simulink model "Regler_opt"  (R2026a)
settings: Solver=ode23s  StartTime=tSim(1)  StopTime=tSim(end)  FixedStep=tStep  EnableMultiTasking=on
values from neighbouring files (symbols this model uses):
  A = [ 0,      1, 0,      0 ... (first row only)    [A4_4.m]    (also in reglerInit.m = [0, 1, 0, 0; reglerInit_fin.m = [0, 1, 0, 0; reglerInit_gain_scheduling.m = [0, 1, 0, 0; reglerInit_opt.m = [0, 1, 0, 0)
  A_grid = zeros(N_ml, 16)    [reglerInit_fin.m]    (also in reglerInit_opt1.m; reglerInit_opt2.m; reglerInit_opt3.m; reglerInit_opt4.m)
  a_lim_large = 3.0    (= 3)    [reglerInit_opt4.m]
  a_lim_medium = 2.6    [reglerInit_opt4.m]
  a_lim_small = 1.4    [reglerInit_opt4.m]
  A_obs = A - L_obs*C    [reglerInit.m]    (also in reglerInit_gain_scheduling.m; reglerInit_opt.m)
  a_ref0 = 0    [reglerInit_fin.m]    (also in reglerInit_opt2.m; reglerInit_opt3.m; reglerInit_opt4.m)
  a_ref_lim = 3.91175    [reglerInit_fin.m]    (also in reglerInit_opt2.m = 3.8; reglerInit_opt3.m = 3.8)
  A_traj = [0, 1, 0 ... (first row only)    [reglerInit_opt.m]    (also in reglerInit_opt1.m)
  B = [0; -30.49; 0; 30.49]    [A4_4.m]    (also in reglerInit.m; reglerInit_fin.m; reglerInit_gain_scheduling.m; reglerInit_opt.m)
  B_obs = [B, L_obs]    [reglerInit.m]    (also in reglerInit_gain_scheduling.m; reglerInit_opt.m)
  B_traj = [0 ... (first row only)    [reglerInit_opt.m]    (also in reglerInit_opt1.m)
  C = [1 0 0 0 ... (first row only)    [reglerInit.m]    (also in reglerInit_fin.m; reglerInit_gain_scheduling.m; reglerInit_opt.m; reglerInit_opt1.m)
  C_obs = eye(4)    [reglerInit.m]    (also in reglerInit_gain_scheduling.m; reglerInit_opt.m)
  C_traj = eye(3)    [reglerInit_opt.m]    (also in reglerInit_opt1.m)
  d_capture_full = 0.03    [reglerInit_opt3.m]    (also in reglerInit_opt4.m = 0.1)
  d_capture_start = 0.10    (= 0.1)    [reglerInit_opt3.m]    (also in reglerInit_opt4.m = 0.35)
  d_large = 1.18779    [reglerInit_fin.m]    (also in reglerInit_opt2.m = 1.3; reglerInit_opt3.m = 1.3; reglerInit_opt4.m = 1.2)
  D_obs = zeros(4,3)    [reglerInit.m]    (also in reglerInit_gain_scheduling.m; reglerInit_opt.m)
  d_small = 0.5719    [reglerInit_fin.m]    (also in reglerInit_opt2.m = 0.45; reglerInit_opt3.m = 0.45; reglerInit_opt4.m = 0.35)
  D_traj = zeros(3,1)    [reglerInit_opt.m]    (also in reglerInit_opt1.m)
  d_traj_capture = 0.35    [reglerInit_opt4.m]
  ff_gain = 0.942931    [reglerInit_fin.m]    (also in reglerInit_opt.m = 1; reglerInit_opt1.m = 1; reglerInit_opt2.m = 1; reglerInit_opt3.m = 1)
  g = 9.81    [reglerInit_fin.m]    (also in reglerInit_opt.m; reglerInit_opt1.m; reglerInit_opt2.m; reglerInit_opt3.m)
  gamma_phi = 0.195386    [reglerInit_fin.m]    (also in reglerInit_opt2.m = 0.3; reglerInit_opt3.m = 0.3; reglerInit_opt4.m = 0)
  j_lim_large = 14.0    (= 14)    [reglerInit_opt4.m]
  j_lim_medium = 12.0    (= 12)    [reglerInit_opt4.m]
  j_lim_small = 6.0    (= 6)    [reglerInit_opt4.m]
  j_ref_lim = 24.6332    [reglerInit_fin.m]    (also in reglerInit_opt2.m = 20; reglerInit_opt3.m = 20)
  K_capture_grid = zeros(N_ml, 4)    [reglerInit_opt3.m]    (also in reglerInit_opt4.m)
  K_drive_grid = zeros(N_ml, 4)    [reglerInit_opt3.m]    (also in reglerInit_opt4.m)
  K_grid = zeros(N_ml, 4)    [reglerInit_fin.m]    (also in reglerInit_opt1.m; reglerInit_opt2.m)
  K_lqr = lqr(A, B, Q_lqr, R_lqr)    [reglerInit_fin.m]    (also in reglerInit_opt.m; reglerInit_opt1.m; reglerInit_opt2.m; reglerInit_opt3.m)
  k_r = 7.2e-3    (= 0.0072)    [reglerInit_fin.m]    (also in reglerInit_opt.m; reglerInit_opt1.m; reglerInit_opt2.m; reglerInit_opt3.m)
  kd_traj_capture = 7.0    (= 7)    [reglerInit_opt4.m]
  kp_traj_capture = 16.0    (= 16)    [reglerInit_opt4.m]
  l = 1.0    (= 1)    [reglerInit_opt3.m]    (also in reglerInit_opt4.m)
  L_grid = zeros(N_ml, 8)    [reglerInit_fin.m]    (also in reglerInit_opt1.m; reglerInit_opt2.m; reglerInit_opt3.m; reglerInit_opt4.m)
  L_obs = place(A', C', obs_poles)'    [reglerInit.m]    (also in reglerInit_fin.m; reglerInit_gain_scheduling.m; reglerInit_opt.m; reglerInit_opt1.m)
  M_ff_max = 0.39    [reglerInit_fin.m]    (also in reglerInit_opt.m = 0.34; reglerInit_opt1.m = 0.34; reglerInit_opt2.m = 0.34; reglerInit_opt3.m = 0.34)
  M_max_total = 0.4    [reglerInit.m]    (also in reglerInit_fin.m; reglerInit_gain_scheduling.m; reglerInit_opt.m; reglerInit_opt1.m)
  m_s = 0.8    [reglerInit_fin.m]    (also in reglerInit_opt.m; reglerInit_opt1.m; reglerInit_opt2.m; reglerInit_opt3.m)
  ml_grid = linspace(1, 5, 17)    [reglerInit_fin.m]    (also in reglerInit_opt1.m; reglerInit_opt2.m; reglerInit_opt3.m; reglerInit_opt4.m)
  omega_ref_large = 2.08014    [reglerInit_fin.m]    (also in reglerInit_opt2.m = 2; reglerInit_opt3.m = 2)
  omega_ref_medium = 3.57058    [reglerInit_fin.m]    (also in reglerInit_opt2.m = 3.3; reglerInit_opt3.m = 3.3)
  omega_ref_small = 3.92272    [reglerInit_fin.m]    (also in reglerInit_opt2.m = 3.3; reglerInit_opt3.m = 3.3)
  phi_ref_lim = deg2rad(35)    [reglerInit_fin.m]    (also in reglerInit_opt2.m = deg2rad(18); reglerInit_opt3.m = deg2rad(18); reglerInit_opt4.m = deg2rad(10))
  phi_slow_1 = deg2rad(26.517)    [reglerInit_fin.m]    (also in reglerInit_opt2.m = deg2rad(28); reglerInit_opt3.m = deg2rad(28); reglerInit_opt4.m = deg2rad(28))
  phi_slow_2 = deg2rad(30.8674)    [reglerInit_fin.m]    (also in reglerInit_opt2.m = deg2rad(36); reglerInit_opt3.m = deg2rad(36); reglerInit_opt4.m = deg2rad(36))
  phidot_ref_lim = 1.6    [reglerInit_fin.m]    (also in reglerInit_opt2.m = 0.8; reglerInit_opt3.m = 0.8; reglerInit_opt4.m = 0)
  r_wheel = 0.041    [reglerInit_fin.m]    (also in reglerInit_opt.m; reglerInit_opt1.m; reglerInit_opt2.m; reglerInit_opt3.m)
  T_a_ref = 0.12    [reglerInit_opt4.m]
  v_lim_large = 2.3    [reglerInit_opt4.m]
  v_lim_medium = 1.8    [reglerInit_opt4.m]
  v_lim_small = 0.75    [reglerInit_opt4.m]
  v_ref0 = 0    [reglerInit_fin.m]    (also in reglerInit_opt2.m; reglerInit_opt3.m; reglerInit_opt4.m)
  x_ref0 = 0    [reglerInit_fin.m]    (also in reglerInit_opt2.m; reglerInit_opt3.m; reglerInit_opt4.m)
  xhat0 = [0, 0, 0, 0]    [reglerInit.m]    (also in reglerInit_fin.m = [0; 0; 0; 0]; reglerInit_gain_scheduling.m; reglerInit_opt.m = [0; 0; 0; 0]; reglerInit_opt1.m = [0; 0; 0; 0])
  xtraj0 = [0; 0; 0]    [reglerInit_opt.m]    (also in reglerInit_opt1.m)
settings Model: Creator=Henning Schlüter  LastModifiedBy=louis
settings DataIOCC: SignalLoggingSaveFormat=ModelDataLogs
settings DebuggingCC: UnderspecifiedInitializationDetection=Classic  PregeneratedLibrarySubsystemCodeDiagnostic=none
settings HardwareCC: ProdHWDeviceType=32-bit Generic
settings GRTTargetCC: CombineOutputUpdateFcns=off  GRTInterface=on

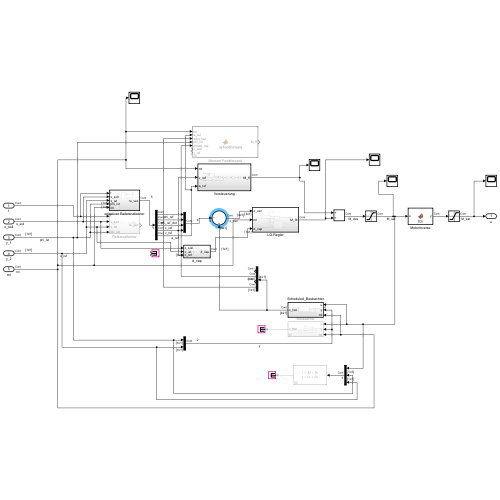
[thumbnail: Simulink's stored preview of the top-level diagram]
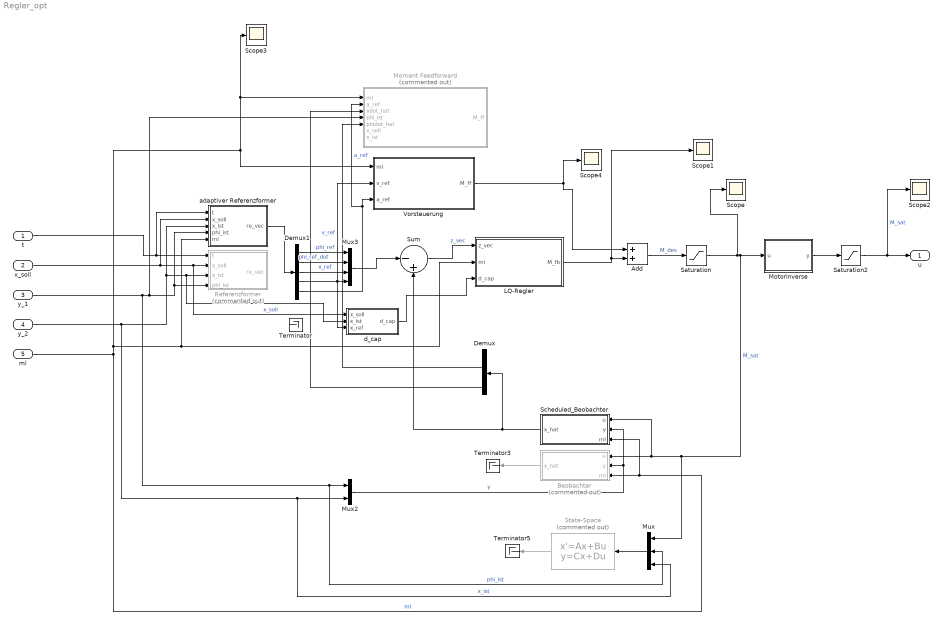
== system Regler_opt ==
  t : Inport  OutDataTypeStr=double  PortDimensions=1  SampleTime=0
  "x_soll " : Inport  Port=2  OutDataTypeStr=double  PortDimensions=1  SampleTime=0
  y_1 : Inport  Port=3  OutDataTypeStr=double  PortDimensions=[1 1]  SampleTime=0
  y_2 : Inport  Port=4  OutDataTypeStr=double  PortDimensions=[1 1]  SampleTime=0
  ml : Inport  Port=5  OutDataTypeStr=double  PortDimensions=1  SampleTime=0
  Add : Sum
  Beobachter : Subsystem  Commented=on
  Demux : Demux
  Demux1 : Demux  Outputs=5
  LQ-Regler : Subsystem
  Moment Feedforward : MATLAB Function  Commented=on  TreatAsAtomicUnit=on
  Motorinverse : MATLAB Function  TreatAsAtomicUnit=on
  Mux : Mux  Inputs=3
  Mux2 : Mux  Inputs=2
  Mux3 : Mux
  Referenzformer : Subsystem  Commented=on
  Saturation : Saturate  UpperLimit=M_max_total  LowerLimit=-M_max_total
  Saturation2 : Saturate  UpperLimit=100  LowerLimit=-100
  Scheduled_Beobachter : Subsystem
  Scope{,1..4} (5 alike) : Scope
      Scope settings: ActiveDisplayYMinimum=-0.49175375586070769  ActiveDisplayYMaximum=-0.20102751095454277
      Scope1 settings: ActiveDisplayYMinimum=-0.094687281937852363  ActiveDisplayYMaximum=1.6990664417619266
      Scope2 settings: ActiveDisplayYMinimum=27.519723000110169  ActiveDisplayYMaximum=88.458122086201712  DataLoggingVariableName=ScopeData2
      Scope3 settings: ActiveDisplayYMinimum=0.60192793931732025  ActiveDisplayYMaximum=5.3638327012220817  DataLoggingVariableName=ScopeData3
      Scope4 settings: ActiveDisplayYMinimum=-0.15043823578049448  ActiveDisplayYMaximum=0.16991782466155569  DataLoggingVariableName=ScopeData6
  State-Space : StateSpace  Commented=on  A=A_obs  B=B_obs  C=C_obs  D=D_obs  InitialCondition=0
  Sum : Sum  Inputs=|-+
  Terminator : Terminator
  Terminator3 : Terminator
  Terminator5 : Terminator
  Vorsteuerung : Subsystem
  adaptiver Referenzformer : Subsystem
  d_cap : Subsystem
  u : Outport  OutDataTypeStr=double  PortDimensions=1  VectorParamsAs1DForOutWhenUnconnected=off
  wires:
  Saturation/1 -> Scheduled_Beobachter/1(u), Beobachter/1(u), Mux/1, Motorinverse/1(u), Scope/1  "M_sat"
  Motorinverse/1(y) -> Saturation2/1
  State-Space/1 -> Terminator5/1
  adaptiver Referenzformer/1(re_vec) -> Demux1/1
  y_2/1 -> Mux/3, Mux2/2, d_cap/2(x_ist), Referenzformer/3(x_ist), adaptiver Referenzformer/3(x_ist)  "x_ist"
  Saturation2/1 -> u/1, Scope2/1  "M_sat"
  Beobachter/1(x_hat) -> Terminator3/1
  Mux/1 -> State-Space/1
  t/1 -> adaptiver Referenzformer/1(t), Referenzformer/1(t)
  Mux2/1 -> Scheduled_Beobachter/2(y), Beobachter/2(y)  "y"
  "x_soll "/1 -> adaptiver Referenzformer/2(x_soll), d_cap/1(x_soll), Referenzformer/2(x_soll)  "x_soll"
  y_1/1 -> Moment Feedforward/4(phi_ist), adaptiver Referenzformer/4(phi_ist), Referenzformer/4(phi_ist), Mux/2, Mux2/1  "phi_ist"
  ml/1 -> LQ-Regler/2(ml), adaptiver Referenzformer/5(ml), Scope3/1, Moment Feedforward/1(ml), Vorsteuerung/1(ml), Scheduled_Beobachter/3(ml), Beobachter/3(ml)  "ml"
  Demux1/1 -> Mux3/1  "phi_ref"
  Demux1/2 -> Mux3/2  "phi_ref_dot"
  Demux1/3 -> Mux3/3  "x_ref"
  Demux1/4 -> d_cap/3(x_ref), Vorsteuerung/2(v_ref), Mux3/4  "v_ref"
  Mux3/1 -> Sum/1
  Add/1 -> Saturation/1  "M_des"
  Vorsteuerung/1(M_ff) -> Add/1, Scope4/1
  Demux1/5 -> Vorsteuerung/3(a_ref), Moment Feedforward/2(a_ref)  "a_ref"
  LQ-Regler/1(M_fb) -> Scope1/1, Add/2
  Sum/1 -> LQ-Regler/1(z_vec)  "z_vec"
  Scheduled_Beobachter/1(x_hat) -> Demux/1, Sum/2
  d_cap/1(d_cap) -> LQ-Regler/3(d_cap)
  Demux/2 -> Moment Feedforward/5(phidot_hat)
  Demux/4 -> Moment Feedforward/3(xdot_hat)

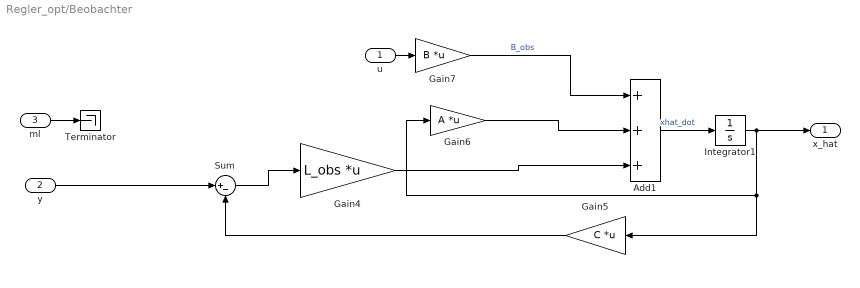
== system Regler_opt/Beobachter ==
  u : Inport
  y : Inport  Port=2
  ml : Inport  Port=3
  Add1 : Sum  Inputs=+++
  Gain4 : Gain  Gain=L_obs  Multiplication=Matrix(K*u)
  Gain5 : Gain  Gain=C  Multiplication=Matrix(K*u)
  Gain6 : Gain  Gain=A  Multiplication=Matrix(K*u)
  Gain7 : Gain  Gain=B  Multiplication=Matrix(K*u)
  Integrator1 : Integrator  InitialCondition=xhat0
  Sum : Sum  Inputs=|+-
  Terminator : Terminator
  x_hat : Outport
  wires:
  u/1 -> Gain7/1
  Gain7/1 -> Add1/1  "B_obs"
  Add1/1 -> Integrator1/1  "xhat_dot"
  Integrator1/1 -> Gain6/1, Gain5/1, x_hat/1
  Gain6/1 -> Add1/2
  Gain4/1 -> Add1/3
  ml/1 -> Terminator/1
  y/1 -> Sum/1
  Gain5/1 -> Sum/2
  Sum/1 -> Gain4/1

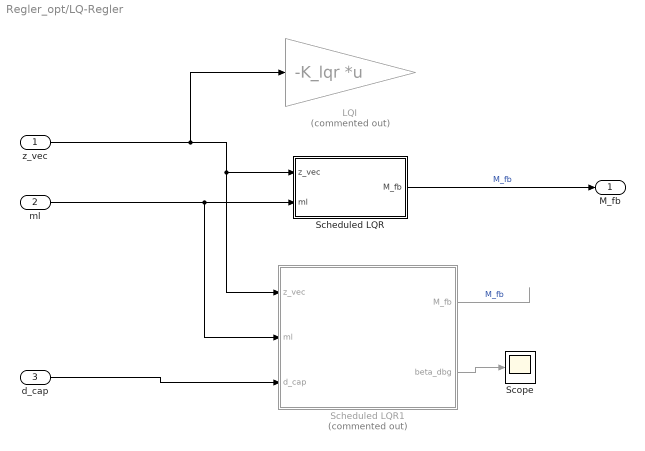
== system Regler_opt/LQ-Regler ==
  z_vec : Inport
  ml : Inport  Port=2
  d_cap : Inport  Port=3
  LQI : Gain  Commented=on  Gain=-K_lqr  Multiplication=Matrix(K*u)
  Scheduled LQR : MATLAB Function  TreatAsAtomicUnit=on
  Scheduled LQR1 : MATLAB Function  Commented=on  TreatAsAtomicUnit=on
  Scope : Scope
      settings: ActiveDisplayYMinimum=0.035956044230071649  ActiveDisplayYMaximum=0.99107395840317047  DataLoggingVariableName=ScopeData8
  M_fb : Outport
  wires:
  z_vec/1 -> LQI/1, Scheduled LQR1/1(z_vec), Scheduled LQR/1(z_vec)
  Scheduled LQR1/1(M_fb) -> ?  "M_fb"
  ml/1 -> Scheduled LQR1/2(ml), Scheduled LQR/2(ml)
  Scheduled LQR1/2(beta_dbg) -> Scope/1
  d_cap/1 -> Scheduled LQR1/3(d_cap)
  Scheduled LQR/1(M_fb) -> M_fb/1  "M_fb"

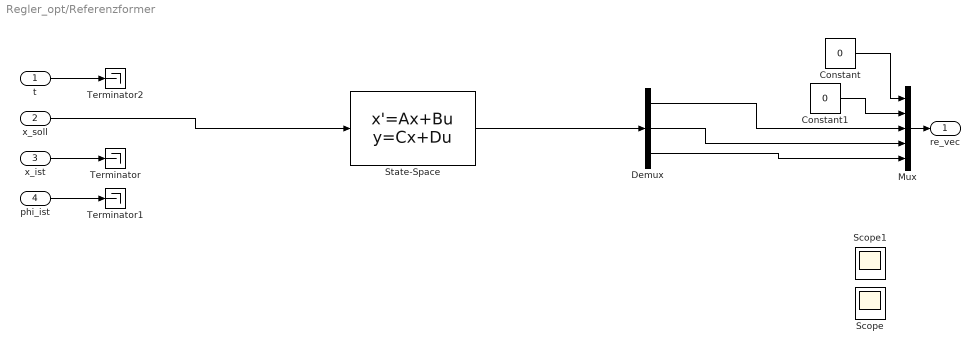
== system Regler_opt/Referenzformer ==
  t : Inport
  x_soll : Inport  Port=2
  x_ist : Inport  Port=3
  phi_ist : Inport  Port=4
  Constant : Constant  Value=0
  Constant1 : Constant  Value=0
  Demux : Demux  Outputs=3
  Mux : Mux  Inputs=5
  Scope : Scope
      settings: ActiveDisplayYMinimum=-1.648469938874336  ActiveDisplayYMaximum=0.49292600283554422  DataLoggingVariableName=ScopeData4
  Scope1 : Scope
      settings: ActiveDisplayYMinimum=-0.15489744027848928  ActiveDisplayYMaximum=0.17747491637319093  DataLoggingVariableName=ScopeData5
  State-Space : StateSpace  A=A_traj  B=B_traj  C=C_traj  D=D_traj  InitialCondition=xtraj0
  Terminator : Terminator
  Terminator1 : Terminator
  Terminator2 : Terminator
  re_vec : Outport
  wires:
  x_soll/1 -> State-Space/1
  State-Space/1 -> Demux/1
  Mux/1 -> re_vec/1
  Demux/1 -> Mux/3
  Demux/2 -> Mux/4
  Constant1/1 -> Mux/2
  Constant/1 -> Mux/1
  t/1 -> Terminator2/1
  phi_ist/1 -> Terminator1/1
  x_ist/1 -> Terminator/1
  Demux/3 -> Mux/5

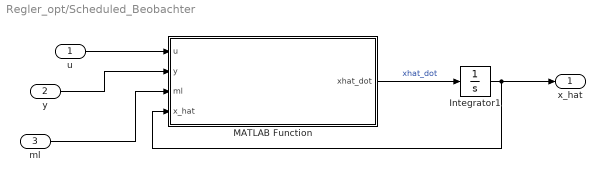
== system Regler_opt/Scheduled_Beobachter ==
  u : Inport
  y : Inport  Port=2
  ml : Inport  Port=3
  Integrator1 : Integrator  InitialCondition=xhat0
  MATLAB Function : MATLAB Function  TreatAsAtomicUnit=on
  x_hat : Outport
  wires:
  u/1 -> MATLAB Function/1(u)
  MATLAB Function/1(xhat_dot) -> Integrator1/1  "xhat_dot"
  Integrator1/1 -> MATLAB Function/4(x_hat), x_hat/1
  ml/1 -> MATLAB Function/3(ml)
  y/1 -> MATLAB Function/2(y)

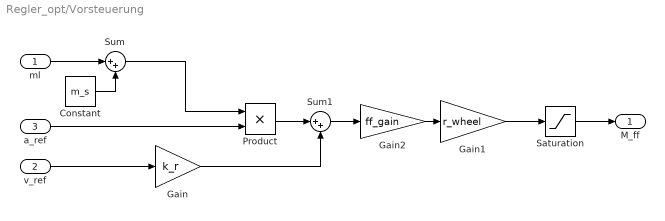
== system Regler_opt/Vorsteuerung ==
  ml : Inport
  v_ref : Inport  Port=2
  a_ref : Inport  Port=3
  Constant : Constant  Value=m_s
  Gain : Gain  Gain=k_r
  Gain1 : Gain  Gain=r_wheel
  Gain2 : Gain  Gain=ff_gain
  Product : Product
  Saturation : Saturate  UpperLimit=M_ff_max  LowerLimit=-M_ff_max
  Sum : Sum  Inputs=|++
  Sum1 : Sum  Inputs=|++
  M_ff : Outport
  wires:
  ml/1 -> Sum/1
  a_ref/1 -> Product/2
  Saturation/1 -> M_ff/1
  v_ref/1 -> Gain/1
  Constant/1 -> Sum/2
  Sum/1 -> Product/1
  Gain1/1 -> Saturation/1
  Gain2/1 -> Gain1/1
  Sum1/1 -> Gain2/1
  Product/1 -> Sum1/1
  Gain/1 -> Sum1/2

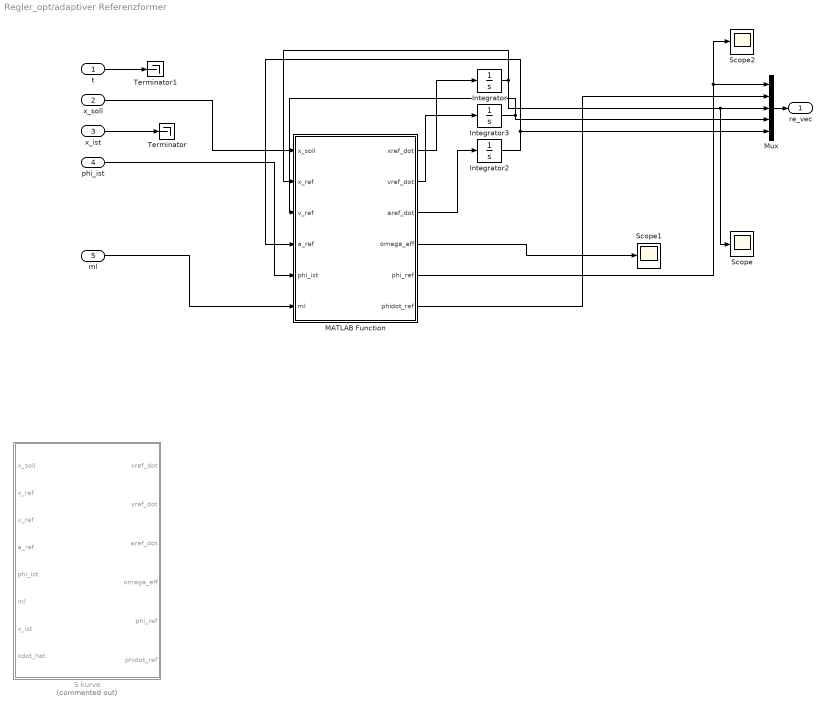
== system Regler_opt/adaptiver Referenzformer ==
  t : Inport
  x_soll : Inport  Port=2
  x_ist : Inport  Port=3
  phi_ist : Inport  Port=4
  ml : Inport  Port=5
  Integrator : Integrator  InitialCondition=x_ref0
  Integrator2 : Integrator  InitialCondition=a_ref0
  Integrator3 : Integrator  InitialCondition=v_ref0
  MATLAB Function : MATLAB Function  TreatAsAtomicUnit=on
  Mux : Mux  Inputs=5
  S kurve : MATLAB Function  Commented=on  TreatAsAtomicUnit=on
  Scope : Scope
      settings: ActiveDisplayYMinimum=-1.648469938874336  ActiveDisplayYMaximum=0.49292600283554422  DataLoggingVariableName=ScopeData4
  Scope1 : Scope
      settings: ActiveDisplayYMinimum=-0.15489744027848928  ActiveDisplayYMaximum=0.17747491637319093  DataLoggingVariableName=ScopeData5
  Scope2 : Scope
      settings: ActiveDisplayYMinimum=-1.648469938874336  ActiveDisplayYMaximum=0.49292600283554422  DataLoggingVariableName=ScopeData7
  Terminator : Terminator
  Terminator1 : Terminator
  re_vec : Outport
  wires:
  Mux/1 -> re_vec/1
  t/1 -> Terminator1/1
  phi_ist/1 -> MATLAB Function/5(phi_ist)
  x_ist/1 -> Terminator/1
  ml/1 -> MATLAB Function/6(ml)
  x_soll/1 -> MATLAB Function/1(x_soll)
  MATLAB Function/2(vref_dot) -> Integrator3/1
  MATLAB Function/1(xref_dot) -> Integrator/1
  MATLAB Function/3(aref_dot) -> Integrator2/1
  Integrator/1 -> MATLAB Function/2(x_ref), Scope/1, Mux/3
  Integrator3/1 -> MATLAB Function/3(v_ref), Mux/4
  Integrator2/1 -> MATLAB Function/4(a_ref), Mux/5
  MATLAB Function/6(phidot_ref) -> Mux/2
  MATLAB Function/5(phi_ref) -> Scope2/1, Mux/1
  MATLAB Function/4(omega_eff) -> Scope1/1

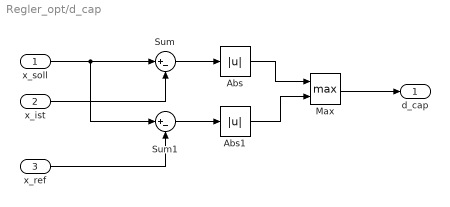
== system Regler_opt/d_cap ==
  x_soll : Inport
  x_ist : Inport  Port=2
  x_ref : Inport  Port=3
  Abs : Abs  SaturateOnIntegerOverflow=off
  Abs1 : Abs  SaturateOnIntegerOverflow=off
  Max : MinMax  Function=max  Inputs=2
  Sum : Sum  Inputs=|+-
  Sum1 : Sum  Inputs=|+-
  d_cap : Outport
  wires:
  x_soll/1 -> Sum1/1, Sum/1
  x_ist/1 -> Sum/2
  x_ref/1 -> Sum1/2
  Sum/1 -> Abs/1
  Sum1/1 -> Abs1/1
  Abs/1 -> Max/1
  Abs1/1 -> Max/2
  Max/1 -> d_cap/1

== matlab function Regler_opt/Scheduled_Beobachter/MATLAB Function ==
  data: u input double size=1; xhat_dot output double size=[4 1]; y input double size=2; ml input double size=1; x_hat input double size=4; ml_grid parameter double size=[1 17]; A_grid parameter double size=[17 16]; L_grid parameter double size=[17 8]; B parameter double size=[4 1]; C parameter double size=[2 4]
function xhat_dot = ScheduledObserver(u, y, ml, x_hat, ml_grid, A_grid, L_grid, B, C)
%#codegen

xhat_dot = zeros(4,1);

% Eingänge robust lesen
u  = double(u(1));
ml = double(ml(1));

y1 = double(y(1));
y2 = double(y(2));

xh1 = double(x_hat(1));
xh2 = double(x_hat(2));
xh3 = double(x_hat(3));
xh4 = double(x_hat(4));

% Scheduling-Index und Interpolation
if ml <= ml_grid(1)
    idx = 1;
    alpha = 0.0;

elseif ml >= ml_grid(end)
    idx = length(ml_grid) - 1;
    alpha = 1.0;

else
    n = length(ml_grid);
    idx = 1;

    for i = 1:n-1
        if ml >= ml_grid(i) && ml <= ml_grid(i+1)
            idx = i;
            break;
        end
    end

    alpha = (ml - ml_grid(idx)) / (ml_grid(idx+1) - ml_grid(idx));
end

% A und L interpolieren
Arow = zeros(1,16);
Lrow = zeros(1,8);

for j = 1:16
    Arow(j) = (1-alpha)*A_grid(idx,j) + alpha*A_grid(idx+1,j);
end

for j = 1:8
    Lrow(j) = (1-alpha)*L_grid(idx,j) + alpha*L_grid(idx+1,j);
end

A_ml = reshape(Arow, 4, 4);
L_ml = reshape(Lrow, 4, 2);

xv = [xh1; xh2; xh3; xh4];
yv = [y1; y2];

% Beobachtergleichung:
% xhat_dot = A(ml)*xhat + B*u + L(ml)*(y - C*xhat)
y_hat = C * xv;
e_y = yv - y_hat;

xhat_dot = A_ml*xv + B*u + L_ml*e_y;

== matlab function Regler_opt/adaptiver Referenzformer/MATLAB Function ==
  data: x_soll input double size=1; xref_dot output double size=1; x_ref input double size=1; v_ref input double size=1; a_ref input double size=1; phi_ist input double size=1; ml input double size=1; vref_dot output double size=1; aref_dot output double size=1; omega_eff output double size=1; phi_ref output double size=1; phidot_ref_lim parameter double size=[1 1]; g parameter double size=[1 1]; gamma_phi parameter double size=[1 1]; phi_ref_lim parameter double size=[1 1]; j_ref_lim parameter double size=[1 1]; a_ref_lim parameter double size=[1 1]; phi_slow_2 parameter double size=[1 1]; phi_slow_1 parameter double size=[1 1]; d_small parameter double size=[1 1]; d_large parameter double size=[1 1]; omega_ref_small parameter double size=[1 1]; omega_ref_medium parameter double size=[1 1]; omega_ref_large parameter double size=[1 1]; phidot_ref output double size=1
function [xref_dot, vref_dot, aref_dot, omega_eff, phi_ref, phidot_ref] = AdaptiveTrajDyn(x_soll, x_ref, v_ref, a_ref, phi_ist, ml, phidot_ref_lim, g, gamma_phi, phi_ref_lim, j_ref_lim, a_ref_lim, phi_slow_2, phi_slow_1, d_small, d_large, omega_ref_small, omega_ref_medium, omega_ref_large)
%#codegen

% Eingänge robust als Skalare lesen
x_soll  = double(x_soll(1));
x_ref   = double(x_ref(1));
v_ref   = double(v_ref(1));
a_ref   = double(a_ref(1));
phi_ist = double(phi_ist(1));
ml      = double(ml(1));

% Outputs explizit initialisieren
xref_dot   = 0.0;
vref_dot   = 0.0;
aref_dot   = 0.0;
omega_eff  = 0.0;
phi_ref    = 0.0;
phidot_ref = 0.0;

% Abstand zwischen interner Referenz und Soll
d = abs(x_soll - x_ref);

% Adaptive Wahl von omega
if d > d_large
    omega_eff = omega_ref_large;
elseif d > d_small
    omega_eff = omega_ref_medium;
else
    omega_eff = omega_ref_small;
end

% Massenabhängige leichte Anpassung
if ml > 4.0
    omega_eff = 0.90 * omega_eff;
elseif ml < 1.5
    omega_eff = 1.05 * omega_eff;
end

% Sicherheitsreduktion bei großem Pendelausschlag
phi_abs = abs(phi_ist);

if phi_abs > phi_slow_2
    omega_eff = 0.55 * omega_eff;
elseif phi_abs > phi_slow_1
    omega_eff = 0.75 * omega_eff;
end

% Schutz gegen numerisch unguenstige Werte
if omega_eff < 0.2
    omega_eff = 0.2;
elseif omega_eff > 8.0
    omega_eff = 8.0;
end

% Kontinuierlicher Filter 3. Ordnung:
% x''' = omega^3*(x_soll-x_ref) - 3*omega^2*v_ref - 3*omega*a_ref
j_cmd = omega_eff * omega_eff * omega_eff * (x_soll - x_ref) ...
      - 3.0 * omega_eff * omega_eff * v_ref ...
      - 3.0 * omega_eff * a_ref;

% Jerk-Begrenzung
if j_cmd > j_ref_lim
    j_cmd = j_ref_lim;
elseif j_cmd < -j_ref_lim
    j_cmd = -j_ref_lim;
end

% Beschleunigungsbegrenzung
if a_ref > a_ref_lim && j_cmd > 0.0
    j_cmd = 0.0;
elseif a_ref < -a_ref_lim && j_cmd < 0.0
    j_cmd = 0.0;
end

% Integratordynamik
xref_dot = v_ref;
vref_dot = a_ref;
aref_dot = j_cmd;

% Partielle Pendelreferenz
phi_ref = gamma_phi * (-a_ref / g);

if phi_ref > phi_ref_lim
    phi_ref = phi_ref_lim;
elseif phi_ref < -phi_ref_lim
    phi_ref = -phi_ref_lim;
end

% Für den ersten Test bewusst ruhig halten
phidot_ref = 0.0;

== matlab function Regler_opt/LQ-Regler/Scheduled LQR1 ==
  data: z_vec input double size=4; M_fb output double size=1; ml input double size=1; beta_dbg output; d_cap input double size=1; ml_grid parameter size=[1 17]; K_drive_grid parameter size=[17 4]; K_capture_grid parameter size=[17 4]; d_capture_start parameter size=[1 1]; d_capture_full parameter size=[1 1]
function [M_fb, beta_dbg] = ScheduledLQR_DriveCapture(z_vec, ml, d_cap, ml_grid, K_drive_grid, K_capture_grid, d_capture_start, d_capture_full)
%#codegen

M_fb = 0.0;
beta_dbg = 0.0;

ml = double(ml(1));
d_cap = double(d_cap(1));

z1 = double(z_vec(1));
z2 = double(z_vec(2));
z3 = double(z_vec(3));
z4 = double(z_vec(4));

n = length(ml_grid);

idx = 1;
alpha = 0.0;

% Massenintervall suchen
if ml <= ml_grid(1)
    idx = 1;
    alpha = 0.0;

elseif ml >= ml_grid(n)
    idx = n - 1;
    alpha = 1.0;

else
    for i = 1:n-1
        if ml >= ml_grid(i) && ml <= ml_grid(i+1)
            idx = i;
            alpha = (ml - ml_grid(i)) / (ml_grid(i+1) - ml_grid(i));
            break;
        end
    end
end

% Drive-Gain interpolieren
Kd1 = (1.0-alpha)*K_drive_grid(idx,1) + alpha*K_drive_grid(idx+1,1);
Kd2 = (1.0-alpha)*K_drive_grid(idx,2) + alpha*K_drive_grid(idx+1,2);
Kd3 = (1.0-alpha)*K_drive_grid(idx,3) + alpha*K_drive_grid(idx+1,3);
Kd4 = (1.0-alpha)*K_drive_grid(idx,4) + alpha*K_drive_grid(idx+1,4);

% Capture-Gain interpolieren
Kc1 = (1.0-alpha)*K_capture_grid(idx,1) + alpha*K_capture_grid(idx+1,1);
Kc2 = (1.0-alpha)*K_capture_grid(idx,2) + alpha*K_capture_grid(idx+1,2);
Kc3 = (1.0-alpha)*K_capture_grid(idx,3) + alpha*K_capture_grid(idx+1,3);
Kc4 = (1.0-alpha)*K_capture_grid(idx,4) + alpha*K_capture_grid(idx+1,4);

% Drive/Capture-Mischung
if d_cap >= d_capture_start
    beta = 0.0;
elseif d_cap <= d_capture_full
    beta = 1.0;
else
    den = d_capture_start - d_capture_full;
    if den < 1e-6
        den = 1e-6;
    end

    beta = (d_capture_start - d_cap) / den;

    % Smoothstep: vermeidet harten Gain-Knick
    beta = beta * beta * (3.0 - 2.0 * beta);
end

beta_dbg = beta;

% Gemischter Gain
K1 = (1.0-beta)*Kd1 + beta*Kc1;
K2 = (1.0-beta)*Kd2 + beta*Kc2;
K3 = (1.0-beta)*Kd3 + beta*Kc3;
K4 = (1.0-beta)*Kd4 + beta*Kc4;

% Rückführung
M_fb = -(K1*z1 + K2*z2 + K3*z3 + K4*z4);

== matlab function Regler_opt/adaptiver Referenzformer/S kurve ==
  data: x_soll input double size=1; xref_dot output double size=1; x_ref input double size=1; v_ref input double size=1; a_ref input double size=1; phi_ist input double size=1; ml input double size=1; vref_dot output double size=1; aref_dot output double size=1; omega_eff output double size=1; phi_ref output double size=1; phidot_ref output double size=1; v_lim_large parameter double size=[1 1]; a_lim_large parameter double size=[1 1]; j_lim_large parameter double size=[1 1]; v_lim_medium parameter double size=[1 1]; a_lim_medium parameter double size=[1 1]; j_lim_medium parameter double size=[1 1]; v_lim_small parameter double size=[1 1]; a_lim_small parameter double size=[1 1]; j_lim_small parameter double size=[1 1]; d_large parameter double size=[1 1]; d_small parameter double size=[1 1]; d_traj_capture parameter double size=[1 1]; kp_traj_capture parameter double size=[1 1]; kd_traj_capture parameter double size=[1 1]; T_a_ref parameter double size=[1 1]; phi_slow_1 parameter double size=[1 1]; phi_slow_2 parameter double size=[1 1]; gamma_phi parameter double size=[1 1]; phi_ref_lim parameter double size=[1 1]; phidot_ref_lim parameter double size=[1 1]; g parameter double size=[1 1]; x_ist input double size=1; xdot_hat input double size=1
function [xref_dot, vref_dot, aref_dot, omega_eff, phi_ref, phidot_ref] = AdaptiveTrajDyn(x_soll, x_ref, v_ref, a_ref, phi_ist, ml, v_lim_large, a_lim_large, j_lim_large, v_lim_medium, a_lim_medium, j_lim_medium, v_lim_small, a_lim_small, j_lim_small, d_large, d_small, d_traj_capture, kp_traj_capture, kd_traj_capture, T_a_ref, phi_slow_1, phi_slow_2, gamma_phi, phi_ref_lim, phidot_ref_lim, g, x_ist, xdot_hat)
%#codegen

% Eingänge
x_ist    = double(x_ist(1));
x_soll  = double(x_soll(1));
xdot_hat = double(xdot_hat(1));
x_ref   = double(x_ref(1));
v_ref   = double(v_ref(1));
a_ref   = double(a_ref(1));
phi_ist = double(phi_ist(1));
ml      = double(ml(1));

% Outputs initialisieren
xref_dot   = 0.0;
vref_dot   = 0.0;
aref_dot   = 0.0;
omega_eff  = 0.0;   % hier als Diagnose: a_des
phi_ref    = 0.0;
phidot_ref = 0.0;

e = x_soll - x_ref;
d = abs(e);

% Richtungswahl
dir = sign(e);
if dir == 0.0
    dir = sign(v_ref);
end
if dir == 0.0
    dir = 1.0;
end

% Parameter abhängig von Distanz wählen
if d > d_large
    v_lim = v_lim_large;
    a_lim = a_lim_large;
    j_lim = j_lim_large;
elseif d > d_small
    v_lim = v_lim_medium;
    a_lim = a_lim_medium;
    j_lim = j_lim_medium;
else
    v_lim = v_lim_small;
    a_lim = a_lim_small;
    j_lim = j_lim_small;
end

% Optional: schwere Last etwas vorsichtiger
if ml > 4.0
    a_lim = 0.90 * a_lim;
    j_lim = 0.90 * j_lim;
elseif ml < 1.5
    a_lim = 1.05 * a_lim;
    j_lim = 1.05 * j_lim;
end

% Safety bei Pendelwinkel
phi_abs = abs(phi_ist);

if phi_abs > phi_slow_2
    a_lim = 0.55 * a_lim;
    j_lim = 0.55 * j_lim;
    v_lim = 0.70 * v_lim;
elseif phi_abs > phi_slow_1
    a_lim = 0.75 * a_lim;
    j_lim = 0.75 * j_lim;
    v_lim = 0.85 * v_lim;
end

% Schutz
if a_lim < 0.1
    a_lim = 0.1;
end
if j_lim < 0.5
    j_lim = 0.5;
end
if v_lim < 0.1
    v_lim = 0.1;
end

% Zusätzliche distanzabhängige Begrenzung:
% Verhindert brutale Beschleunigung bei sehr kleinen Wegen.
a_dist_lim = 0.7 + 6.0*d;

if a_lim > a_dist_lim
    a_lim = a_dist_lim;
end

% Passendes Geschwindigkeitslimit zur verbleibenden Strecke
v_dist_lim = sqrt(2.0*a_lim*d + 1e-6);

if v_lim > v_dist_lim
    v_lim = v_dist_lim;
end

% Mindestwerte gegen numerische Probleme
if a_lim < 0.4
    a_lim = 0.4;
end

if v_lim < 0.15
    v_lim = 0.15;
end

% Prüfen, ob wir uns grob in Richtung Ziel bewegen
moving_towards = false;
if abs(v_ref) < 1e-5
    moving_towards = true;
else
    if sign(v_ref) == dir
        moving_towards = true;
    end
end

% Bremsweg
d_stop = (v_ref*v_ref) / (2.0*a_lim + 1e-9);

% Grundentscheidung für a_des
if d < d_traj_capture || d < d_small
    % Nahe am Ziel: PD-Einfangdynamik für die Referenztrajektorie
    a_des = kp_traj_capture * e - kd_traj_capture * v_ref;

    if a_des > a_lim
        a_des = a_lim;
    elseif a_des < -a_lim
        a_des = -a_lim;
    end

else
    if moving_towards
        if d <= d_stop
            % rechtzeitig bremsen
            a_des = -sign(v_ref) * a_lim;
        else
            % beschleunigen
            a_des = dir * a_lim;
        end
    else
        % falls wir uns vom Ziel weg bewegen: abbremsen/umkehren
        a_des = -sign(v_ref) * a_lim;
    end

    % Geschwindigkeitslimit
    if abs(v_ref) > v_lim
        if sign(v_ref) == sign(a_des)
            a_des = -sign(v_ref) * a_lim;
        end
    end
end

%% Sicherheitsbremse anhand realer Schlittenbewegung

e_act = x_soll - x_ist;
d_act = abs(e_act);

dir_act = sign(e_act);
if dir_act == 0.0
    dir_act = -sign(xdot_hat);
end
if dir_act == 0.0
    dir_act = 1.0;
end

moving_to_target = false;
if abs(xdot_hat) < 1e-5
    moving_to_target = true;
else
    if sign(xdot_hat) == dir_act
        moving_to_target = true;
    end
end

% Bremsweg des realen Schlittens
d_stop_act = (xdot_hat*xdot_hat) / (2.0*a_lim + 1e-9);

% Sicherheitsmarge, wächst mit Geschwindigkeit
brake_margin = 0.10 + 0.08*abs(xdot_hat);

if moving_to_target
    if d_stop_act > max(d_act - brake_margin, 0.0)
        % Realer Schlitten hat zu viel Geschwindigkeit Richtung Ziel:
        % Referenzbeschleunigung auf Bremsen setzen.
        a_des = -sign(xdot_hat) * a_lim;
    end
end

%% Rail-Guard gegen Positionsconstraint

x_guard = 2.30;    % etwas vor dem echten Limit 2.45 eingreifen

if x_ist < -x_guard && xdot_hat < 0.0
    % links nah am Rand und weiter nach links unterwegs -> nach rechts bremsen
    a_des = a_lim;
elseif x_ist > x_guard && xdot_hat > 0.0
    % rechts nah am Rand und weiter nach rechts unterwegs -> nach links bremsen
    a_des = -a_lim;
end

% Jerk-begrenztes Nachführen von a_ref nach a_des
j_cmd = (a_des - a_ref) / T_a_ref;

if j_cmd > j_lim
    j_cmd = j_lim;
elseif j_cmd < -j_lim
    j_cmd = -j_lim;
end

% Integratordynamik
xref_dot = v_ref;
vref_dot = a_ref;
aref_dot = j_cmd;

% Diagnoseausgang
omega_eff = a_des;

% Partielle Pendelreferenz aus aktueller Referenzbeschleunigung
phi_ref = gamma_phi * (-a_ref / g);

if phi_ref > phi_ref_lim
    phi_ref = phi_ref_lim;
elseif phi_ref < -phi_ref_lim
    phi_ref = -phi_ref_lim;
end

% Erstmal ruhig lassen
phidot_ref = 0.0;

== matlab function Regler_opt/Motorinverse ==
  data: u input; y output
function y = fcn(u)

y = sign(u(1)/2)*(9.434*abs(u(1)/2))^2*100/3.56;

== matlab function Regler_opt/LQ-Regler/Scheduled LQR ==
  data: z_vec input double size=4; M_fb output double size=1; ml input double size=1; ml_grid parameter double size=17; K_grid parameter double size=[17 4]
function M_fb = ScheduledLQR(z_vec, ml, ml_grid, K_grid)
%#codegen

% Ausgang explizit initialisieren
M_fb = 0.0;

% Eingänge robust lesen
ml = double(ml(1));

z1 = double(z_vec(1));
z2 = double(z_vec(2));
z3 = double(z_vec(3));
z4 = double(z_vec(4));

% ml auf gueltigen Bereich begrenzen
if ml <= ml_grid(1)
    K1 = K_grid(1,1);
    K2 = K_grid(1,2);
    K3 = K_grid(1,3);
    K4 = K_grid(1,4);

elseif ml >= ml_grid(end)
    n = length(ml_grid);
    K1 = K_grid(n,1);
    K2 = K_grid(n,2);
    K3 = K_grid(n,3);
    K4 = K_grid(n,4);

else
    n = length(ml_grid);
    idx = 1;

    for i = 1:n-1
        if ml >= ml_grid(i) && ml <= ml_grid(i+1)
            idx = i;
            break;
        end
    end

    alpha = (ml - ml_grid(idx)) / (ml_grid(idx+1) - ml_grid(idx));

    K1 = (1-alpha)*K_grid(idx,1) + alpha*K_grid(idx+1,1);
    K2 = (1-alpha)*K_grid(idx,2) + alpha*K_grid(idx+1,2);
    K3 = (1-alpha)*K_grid(idx,3) + alpha*K_grid(idx+1,3);
    K4 = (1-alpha)*K_grid(idx,4) + alpha*K_grid(idx+1,4);
end

% LQR Gesetz
M_fb = -(K1*z1 + K2*z2 + K3*z3 + K4*z4);

== matlab function Regler_opt/Moment Feedforward ==
  data: ml input double size=1; a_ref input double size=1; M_ff output double size=1; xdot_hat input double size=1; phi_ist input double size=1; phidot_hat input double size=1; r_wheel parameter double size=[1 1]; m_s parameter double size=[1 1]; g parameter double size=[1 1]; l parameter double size=[1 1]; k_r parameter double size=[1 1]; ff_gain parameter double size=[1 1]; M_ff_max parameter double size=[1 1]; x_soll input double size=1; x_ist input double size=1
function M_ff = NonlinearFeedforward(ml, a_ref, xdot_hat, phi_ist, phidot_hat, r_wheel, m_s, g, l, k_r, ff_gain, M_ff_max, x_soll, x_ist)
%#codegen

M_ff = 0.0;

ml        = double(ml(1));
a_ref     = double(a_ref(1));
xdot_hat  = double(xdot_hat(1));
phi       = double(phi_ist(1));
phidot    = double(phidot_hat(1));

s = sin(phi);
c = cos(phi);

M_raw = r_wheel * ( ...
    (m_s + ml*s*s) * a_ref ...
    - ml*g*s*c ...
    - ml*l*s*phidot*phidot ...
    + k_r*xdot_hat );

M_ff = ff_gain * M_raw;

d_act = abs(x_soll - x_ist);

ff_scale = 1.0;
if d_act < 0.50
    ff_scale = 0.4 + 0.6*(d_act/0.50);
end

M_ff = ff_scale * M_ff;

if M_ff > M_ff_max
    M_ff = M_ff_max;
elseif M_ff < -M_ff_max
    M_ff = -M_ff_max;
end
